simulink model "Antilock_BrackingSystem"  (R2021a)
settings: Solver=VariableStepAuto  StartTime=0.0  StopTime=25  RelTol=1e-3
undefined symbols (not defined in the file or in its folder): g, I, m, R, v0
settings Model: Creator=Davie  LastModifiedBy=Davie

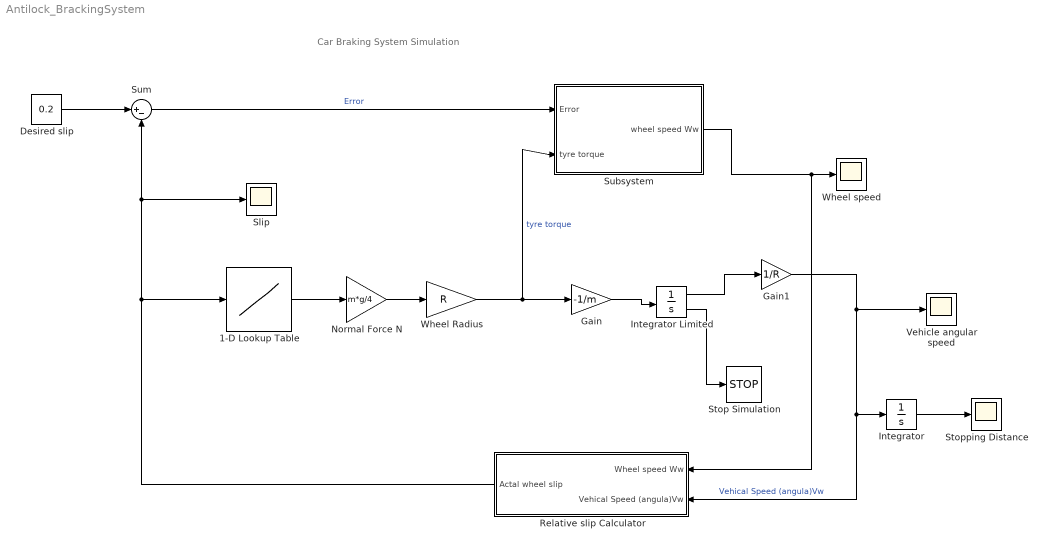
== system Antilock_BrackingSystem ==
  note: Car Braking System Simulation
  1-D Lookup Table : Lookup_n-D  NumberOfTableDimensions=1  BreakpointsForDimension1=[0,0.05,0.1,0.15,0.2,0.25,0.3,0.35,0.4,0.45,0.5,0.55,0.6,0.65,0.7,0.75,0.8,0.85,0.9,0.95,1]  Table=[0,0.4,0.8,0.97,1,0.98,0.96,0.94,0.92,0.9,0.88,0.855,0.83,0.81,0.79,0.77,0.75,0.73,0.72,0.71,0.7]  InternalRulePriority=Speed  RndMeth=Zero  InputSameDT=on
  Desired slip : Constant  Value=0.2
  Gain : Gain  Gain=-1/m
  Gain1 : Gain  Gain=1/R
  Integrator : Integrator
  Integrator Limited : Integrator  InitialCondition=v0  LimitOutput=on  UpperSaturationLimit=1000  LowerSaturationLimit=0  ShowSaturationPort=on
  Normal Force N : Gain  Gain=m*g/4
  "Relative slip Calculator " : Subsystem
  Slip : Scope
  Stop Simulation : Stop
  Stopping Distance : Scope
  Subsystem : Subsystem
  Sum : Sum  Inputs=|+-
  Vehicle angular speed : Scope
  Wheel Radius : Gain  Gain=R
  Wheel speed : Scope
  wires:
  Desired slip/1 -> Sum/1
  1-D Lookup Table/1 -> Normal Force N/1
  Normal Force N/1 -> Wheel Radius/1
  Sum/1 -> Subsystem/1(Error)  "Error"
  Wheel Radius/1 -> Gain/1, Subsystem/2(tyre torque)  "tyre torque"
  Subsystem/1(wheel speed Ww) -> Wheel speed/1, "Relative slip Calculator "/1(Wheel speed Ww)
  Gain/1 -> Integrator Limited/1
  Integrator Limited/1 -> Gain1/1
  Gain1/1 -> "Relative slip Calculator "/2(Vehical Speed (angula)Vw), Integrator/1, Vehicle angular speed/1  "Vehical Speed (angula)Vw"
  Integrator Limited/2 -> Stop Simulation/1
  Integrator/1 -> Stopping Distance/1
  "Relative slip Calculator "/1(Actal wheel slip) -> Sum/2, Slip/1, 1-D Lookup Table/1

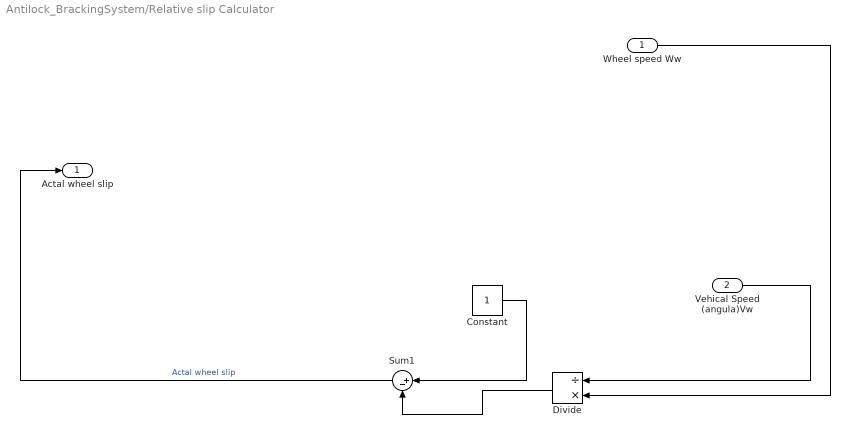
== system Antilock_BrackingSystem/Relative slip Calculator  ==
  Wheel speed Ww : Inport
  Vehical Speed (angula)Vw : Inport  Port=2
  Constant : Constant
  Divide : Product  Inputs=/*
  Sum1 : Sum  Inputs=|+-
  Actal wheel slip : Outport
  wires:
  Constant/1 -> Sum1/1
  Sum1/1 -> Actal wheel slip/1  "Actal wheel slip"
  Vehical Speed (angula)Vw/1 -> Divide/1
  Divide/1 -> Sum1/2
  Wheel speed Ww/1 -> Divide/2

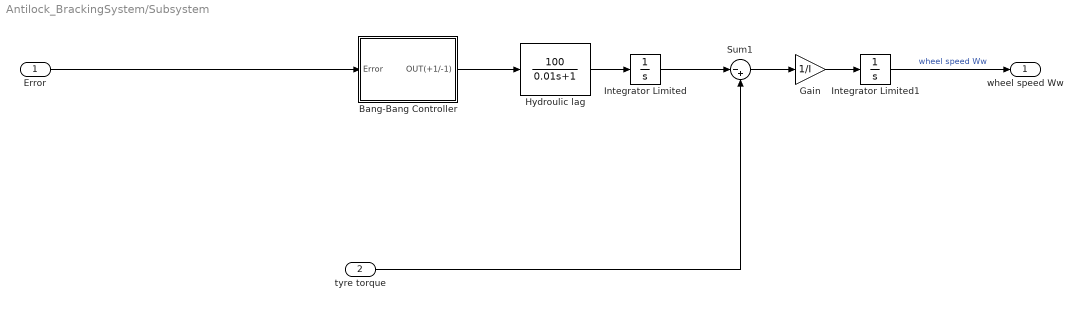
== system Antilock_BrackingSystem/Subsystem ==
  Error : Inport
  tyre torque : Inport  Port=2
  Bang-Bang Controller : Subsystem
  Gain : Gain  Gain=1/I
  Hydroulic lag : TransferFcn  Numerator=[100]  Denominator=[0.01 1]
  Integrator Limited : Integrator  LimitOutput=on  UpperSaturationLimit=1000  LowerSaturationLimit=0
  Integrator Limited1 : Integrator  InitialCondition=v0/R  LimitOutput=on  UpperSaturationLimit=1000  LowerSaturationLimit=0
  Sum1 : Sum  Inputs=|-+
  wheel speed Ww : Outport
  wires:
  tyre torque/1 -> Sum1/2
  Bang-Bang Controller/1(OUT(+1/-1)) -> Hydroulic lag/1
  Integrator Limited/1 -> Sum1/1
  Gain/1 -> Integrator Limited1/1
  Sum1/1 -> Gain/1
  Error/1 -> Bang-Bang Controller/1(Error)
  Hydroulic lag/1 -> Integrator Limited/1
  Integrator Limited1/1 -> wheel speed Ww/1  "wheel speed Ww"

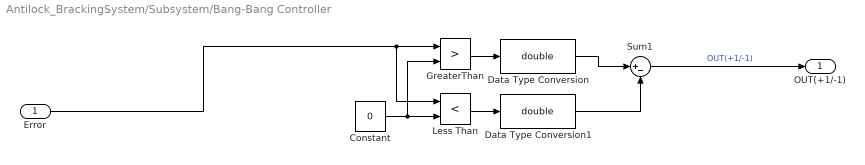
== system Antilock_BrackingSystem/Subsystem/Bang-Bang Controller ==
  Error : Inport
  Constant : Constant  Value=0
  Data Type Conversion : DataTypeConversion  OutDataTypeStr=double  RndMeth=Zero
  Data Type Conversion1 : DataTypeConversion  OutDataTypeStr=double  RndMeth=Zero
  GreaterThan : RelationalOperator  Operator=>  OutDataTypeStr=boolean  RndMeth=Simplest
  Less Than : RelationalOperator  Operator=<  OutDataTypeStr=boolean  RndMeth=Simplest
  Sum1 : Sum  Inputs=|+-
  OUT(+1/-1) : Outport
  wires:
  Data Type Conversion/1 -> Sum1/1
  Data Type Conversion1/1 -> Sum1/2
  GreaterThan/1 -> Data Type Conversion/1
  Less Than/1 -> Data Type Conversion1/1
  Sum1/1 -> OUT(+1/-1)/1  "OUT(+1/-1)"
  Constant/1 -> GreaterThan/2, Less Than/2
  Error/1 -> Less Than/1, GreaterThan/1
